simulink model "PI"  (R2020b)
settings: Solver=VariableStepAuto  StartTime=0.0  StopTime=120  RelTol=1e-3
model workspace (MAT data in the model file):
  Ki = 40
  Kp = 800
  b = 50
  m = 1000
  u = 500
settings Model: DataDictionary=parameter3.sldd  Creator=Puru Gawande  LastModifiedBy=Puru Gawande
settings DataIOCC: SaveOutput=off  SaveTime=off

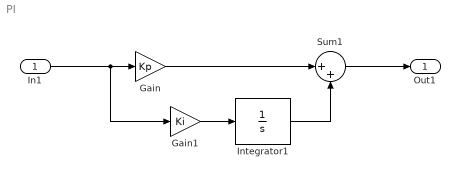
== system PI ==
  In1 : Inport  OutDataTypeStr=double  PortDimensions=1  SampleTime=0
  Gain : Gain  Gain=Kp
  Gain1 : Gain  Gain=Ki
  Integrator1 : Integrator
  Sum1 : Sum  Inputs=|++
  Out1 : Outport  OutDataTypeStr=double  PortDimensions=1  SampleTime=0
  wires:
  Gain1/1 -> Integrator1/1
  In1/1 -> Gain/1, Gain1/1
  Integrator1/1 -> Sum1/2
  Sum1/1 -> Out1/1
  Gain/1 -> Sum1/1
